simulink model "transientStability_R14SP1"  (Simulink 6.1)
settings: Solver=ode4  SolverMode=SingleTasking  StartTime=0.0  StopTime=10  FixedStep=0.01  MaxStep=0.01  RelTol=1e-3  AbsTol=1e-2
undefined symbols (not defined in the file): j, mpc
(part 2 of 3)

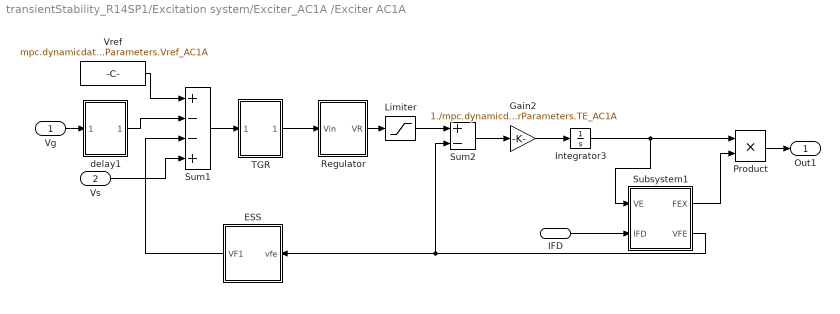
== system transientStability_R14SP1/Excitation system/Exciter_AC1A /Exciter AC1A ==
  Vg : Inport
  Vs : Inport  Port=2
  IFD : Inport  Port=3
  ESS : Subsystem  Orientation=left
  Gain2 : Gain  Gain=1./mpc.dynamicdata.gen_exciterParameters.AC1A_exciterParameters.TE_AC1A  SaturateOnIntegerOverflow=on
  Integrator3 : Integrator  InitialCondition=mpc.dynamicdata.gen_exciterParameters.AC1A_exciterParameters.Ve_AC1A  LimitOutput=on  LowerSaturationLimit=0.01
  Limiter : Saturate  UpperLimit=mpc.dynamicdata.gen_exciterParameters.AC1A_exciterParameters.VRmax_AC1A  LowerLimit=mpc.dynamicdata.gen_exciterParameters.AC1A_exciterParameters.VRmin_AC1A
  Product : Product  SaturateOnIntegerOverflow=on  RndMeth=Zero  InputSameDT=on
  Regulator : Subsystem
  Subsystem1 : Subsystem
  Sum1 : Sum  Inputs=+--+  SaturateOnIntegerOverflow=on  InputSameDT=on
  Sum2 : Sum  Inputs=+-  SaturateOnIntegerOverflow=on  InputSameDT=on
  TGR : Subsystem
  Vref : Constant  Value=mpc.dynamicdata.gen_exciterParameters.AC1A_exciterParameters.Vref_AC1A
  delay1 : Subsystem
  Out1 : Outport
  wires:
  Regulator/1(VR) -> Limiter/1
  Sum1/1 -> TGR/1(Ver)
  TGR/1(Vtgr) -> Regulator/1(Vin)
  Vref/1 -> Sum1/1
  Vs/1 -> Sum1/4
  Product/1 -> Out1/1
  IFD/1 -> Subsystem1/2(IFD)
  Sum2/1 -> Gain2/1
  Limiter/1 -> Sum2/1
  ESS/1(VF1) -> Sum1/3
  Gain2/1 -> Integrator3/1
  Subsystem1/1(FEX) -> Product/2
  Subsystem1/2(VFE) -> ESS/1(vfe), Sum2/2
  Integrator3/1 -> Subsystem1/1(VE), Product/1
  delay1/1(Out1) -> Sum1/2
  Vg/1 -> delay1/1(Vin)

== system transientStability_R14SP1/Excitation system/Exciter_AC1A /Select-AVR ==
  in_1 : Inport
  in_2 : Inport  Port=2
  Switch : Switch  Threshold=1  SaturateOnIntegerOverflow=on  InputSameDT=on
  zeros : Constant  Value=zeros(1,mpc.dynamicdata.extraVariables.nb)
  out_1 : Outport  InitialOutput=0
  wires:
  in_2/1 -> Switch/3
  in_1/1 -> Switch/2
  Switch/1 -> out_1/1
  zeros/1 -> Switch/1

== system transientStability_R14SP1/Excitation system/Exciter_AC4A/DEMUXg2 ==
  In1 : Inport
  Dummy Zeros : Constant  Value=zeros(1,mpc.dynamicdata.extraVariables.nb-size(mpc.dynamicdata.exc_AC4A,1))
  Mux1 : Mux  Inputs="[mpc.dynamicdata.extraVariables.nb-size(mpc.dynamicdata.exc_AC4A,1)  size(mpc.dynamicdata.exc_AC4A,1)]"
  Selector4 : Selector  InputPortWidth=mpc.dynamicdata.extraVariables.nb
  Out1 : Outport
  wires:
  In1/1 -> Mux1/2
  Selector4/1 -> Out1/1
  Dummy Zeros/1 -> Mux1/1
  Mux1/1 -> Selector4/1

== system transientStability_R14SP1/Excitation system/Exciter_AC4A/Exciter_AC4A ==
  Vg : Inport
  Vs : Inport  Port=2
  IFD : Inport  Port=3
  REG : Subsystem
  Saturation : Saturate  UpperLimit=mpc.dynamicdata.gen_exciterParameters.AC4A_exciterParameters.VImax_AC4A  LowerLimit=mpc.dynamicdata.gen_exciterParameters.AC4A_exciterParameters.VImin_AC4A
  Sum1 : Sum  Inputs=+-+  SaturateOnIntegerOverflow=on  InputSameDT=on
  TGR : Subsystem
  Vref1 : Constant  Value=mpc.dynamicdata.gen_exciterParameters.AC4A_exciterParameters.Vref_AC4A
  delay1 : Subsystem
  Out1 : Outport
  wires:
  TGR/1(V3) -> REG/1(In1)
  Vref1/1 -> Sum1/1
  Vs/1 -> Sum1/3
  IFD/1 -> REG/2(IFD)
  REG/1(Out1) -> Out1/1
  Sum1/1 -> Saturation/1
  Saturation/1 -> TGR/1(Ver)
  Vg/1 -> delay1/1(Vin)
  delay1/1(Out1) -> Sum1/2

== system transientStability_R14SP1/Excitation system/Exciter_AC4A/Select-AVR ==
  in_1 : Inport
  in_2 : Inport  Port=2
  Switch : Switch  Threshold=1  SaturateOnIntegerOverflow=on  InputSameDT=on
  zeros : Constant  Value=zeros(1,mpc.dynamicdata.extraVariables.nb)
  out_1 : Outport  InitialOutput=0
  wires:
  in_2/1 -> Switch/3
  in_1/1 -> Switch/2
  Switch/1 -> out_1/1
  zeros/1 -> Switch/1

== system transientStability_R14SP1/Excitation system/Exciter_DC1A/DEMUXg2 ==
  In1 : Inport
  Dummy Zeros : Constant  Value=zeros(1,mpc.dynamicdata.extraVariables.nb-size(mpc.dynamicdata.exc_DC1A,1))
  Mux1 : Mux  Inputs="[mpc.dynamicdata.extraVariables.nb-size(mpc.dynamicdata.exc_DC1A,1)  size(mpc.dynamicdata.exc_DC1A,1)]"
  Selector4 : Selector  InputPortWidth=mpc.dynamicdata.extraVariables.nb
  Out1 : Outport
  wires:
  In1/1 -> Mux1/2
  Selector4/1 -> Out1/1
  Dummy Zeros/1 -> Mux1/1
  Mux1/1 -> Selector4/1

== system transientStability_R14SP1/Excitation system/Exciter_DC1A/Select-AVR ==
  in_1 : Inport
  in_2 : Inport  Port=2
  Switch : Switch  Threshold=1  SaturateOnIntegerOverflow=on  InputSameDT=on
  zeros : Constant  Value=zeros(1,mpc.dynamicdata.extraVariables.nb)
  out_1 : Outport  InitialOutput=0
  wires:
  in_2/1 -> Switch/3
  in_1/1 -> Switch/2
  Switch/1 -> out_1/1
  zeros/1 -> Switch/1

== system transientStability_R14SP1/Excitation system/Exciter_DC1A/Subsystem ==
  Vg : Inport
  Vs : Inport  Port=2
  ESS : Subsystem  Orientation=left
  Gain2 : Gain  Gain=1./mpc.dynamicdata.gen_exciterParameters.DC1A_exciterParameters.TE_DC1A  SaturateOnIntegerOverflow=on
  Integrator3 : Integrator  InitialCondition=mpc.dynamicdata.gen_exciterParameters.DC1A_exciterParameters.Efd0_DC1A
  Regulator : Subsystem
  Saturation : Subsystem  Orientation=left
  Sum1 : Sum  Inputs=+--+  SaturateOnIntegerOverflow=on  InputSameDT=on
  Sum2 : Sum  Inputs=+-  SaturateOnIntegerOverflow=on  InputSameDT=on
  TGR : Subsystem
  Vref : Constant  Value=mpc.dynamicdata.gen_exciterParameters.DC1A_exciterParameters.Vref_DC1A
  delay1 : Subsystem
  Efd : Outport
  wires:
  ESS/1(VF) -> Sum1/3
  Sum1/1 -> TGR/1(Ver)
  TGR/1(V3) -> Regulator/1(Vin)
  Sum2/1 -> Gain2/1
  Gain2/1 -> Integrator3/1
  Saturation/1(VRb) -> Sum2/2
  Integrator3/1 -> Saturation/1(Efd), ESS/1(Efd), Efd/1
  Vs/1 -> Sum1/4
  Vref/1 -> Sum1/1
  delay1/1(Out1) -> Sum1/2
  Vg/1 -> delay1/1(Vin)
  Regulator/1(Out1) -> Sum2/1

== system transientStability_R14SP1/Excitation system/Exciter_ST1A/DEMUXg2 ==
  In1 : Inport
  Dummy Zeros : Constant  Value=zeros(1,mpc.dynamicdata.extraVariables.nb-size(mpc.dynamicdata.exc_ST1A,1))
  Mux1 : Mux  Inputs="[mpc.dynamicdata.extraVariables.nb-size(mpc.dynamicdata.exc_ST1A,1)  size(mpc.dynamicdata.exc_ST1A,1)]"
  Selector4 : Selector  InputPortWidth=mpc.dynamicdata.extraVariables.nb
  Out1 : Outport
  wires:
  In1/1 -> Mux1/2
  Selector4/1 -> Out1/1
  Dummy Zeros/1 -> Mux1/1
  Mux1/1 -> Selector4/1

== system transientStability_R14SP1/Excitation system/Exciter_ST1A/Select-AVR ==
  in_1 : Inport
  in_2 : Inport  Port=2
  Switch : Switch  Threshold=1  SaturateOnIntegerOverflow=on  InputSameDT=on
  zeros : Constant  Value=zeros(1,mpc.dynamicdata.extraVariables.nb)
  out_1 : Outport  InitialOutput=0
  wires:
  in_2/1 -> Switch/3
  in_1/1 -> Switch/2
  Switch/1 -> out_1/1
  zeros/1 -> Switch/1

== system transientStability_R14SP1/Excitation system/Exciter_ST1A/delay1 ==
  Vin : Inport
  Gain : Gain  Gain=1./mpc.dynamicdata.gen_exciterParameters.ST1A_exciterParameters.Tr_ST1A  SaturateOnIntegerOverflow=on
  Integrator2 : Integrator  InitialCondition=mpc.dynamicdata.extraVariables.lfl(mpc.dynamicdata.exc_ST1A(:,1),2)
  Sum : Sum  Inputs=+-  SaturateOnIntegerOverflow=on  InputSameDT=on
  Out1 : Outport
  wires:
  Vin/1 -> Sum/1
  Integrator2/1 -> Sum/2, Out1/1
  Sum/1 -> Gain/1
  Gain/1 -> Integrator2/1

== system transientStability_R14SP1/Excitation system/Exciter_ST1A/exc_ST1A ==
  Vg : Inport
  Vs : Inport  Port=2
  IFD : Inport  Port=3
  ESS : Subsystem  Orientation=left
  Gain2 : Gain  Gain=mpc.dynamicdata.gen_exciterParameters.ST1A_exciterParameters.KLR_ST1A  SaturateOnIntegerOverflow=on
  ILR : Constant  Value=mpc.dynamicdata.gen_exciterParameters.ST1A_exciterParameters.ILR_ST1A
  Limiter : Subsystem
  Rergulator : Subsystem
  Saturation1 : Saturate  UpperLimit=inf  LowerLimit=0
  Sum1 : Sum  Inputs=+-+-  SaturateOnIntegerOverflow=on  InputSameDT=on
  Sum2 : Sum  Inputs=+-  SaturateOnIntegerOverflow=on  InputSameDT=on
  Sum3 : Sum  Inputs=+-  SaturateOnIntegerOverflow=on  InputSameDT=on
  TGR : Subsystem
  Vref1 : Constant  Value=mpc.dynamicdata.gen_exciterParameters.ST1A_exciterParameters.Vref_ST1A
  out_1 : Outport  InitialOutput=0
  wires:
  Vref1/1 -> Sum1/1
  Vs/1 -> Sum1/3
  Rergulator/1(Out1) -> Sum3/1
  Vg/1 -> Sum1/2, Limiter/3(Vt)
  Limiter/1(Out1) -> out_1/1
  ILR/1 -> Sum2/2
  Sum2/1 -> Gain2/1
  Gain2/1 -> Saturation1/1
  Saturation1/1 -> Sum3/2
  IFD/1 -> Sum2/1, Limiter/2(IFD)
  Sum1/1 -> TGR/1(Ver)
  TGR/1(V3) -> Rergulator/1(In1)
  Sum3/1 -> Limiter/1(In1), ESS/1(Efd)
  ESS/1(VF) -> Sum1/4

== system transientStability_R14SP1/Excitation system/Exciter_ST2A/DEMUXg2 ==
  In1 : Inport
  Dummy Zeros : Constant  Value=zeros(1,mpc.dynamicdata.extraVariables.nb-size(mpc.dynamicdata.exc_ST2A,1))
  Mux1 : Mux  Inputs="[mpc.dynamicdata.extraVariables.nb-size(mpc.dynamicdata.exc_ST2A,1)  size(mpc.dynamicdata.exc_ST2A,1)]"
  Selector4 : Selector  InputPortWidth=mpc.dynamicdata.extraVariables.nb
  Out1 : Outport
  wires:
  Mux1/1 -> Selector4/1
  Dummy Zeros/1 -> Mux1/1
  Selector4/1 -> Out1/1
  In1/1 -> Mux1/2

== system transientStability_R14SP1/Excitation system/Exciter_ST2A/ST2A_Exciter ==
  IFD : Inport
  Ia : Inport  Port=2
  Vg : Inport  Port=3
  Vs : Inport  Port=4
  Comp to Mag : ComplexToMagnitudeAngle
  ESS : Subsystem  Orientation=left
  Product4 : Product  SaturateOnIntegerOverflow=on  RndMeth=Zero  InputSameDT=on
  Regulator : Subsystem
  Subsystem : Subsystem
  Sum2 : Sum  Inputs=+--+  SaturateOnIntegerOverflow=on  InputSameDT=on
  Term : Terminator
      settings: Orientation=down
  Vref : Constant  Value=mpc.dynamicdata.gen_exciterParameters.ST2A_exciterParameters.Vref_ST2A
  exciter : Subsystem
  Efd : Outport
  wires:
  Sum2/1 -> Regulator/1(Vin)
  ESS/1(VF) -> Sum2/3
  Vs/1 -> Sum2/4
  Vref/1 -> Sum2/1
  exciter/1(Out1) -> ESS/1(EFD), Efd/1
  IFD/1 -> Subsystem/2("IFD ")
  Ia/1 -> Subsystem/3(Ia)
  Subsystem/1(VB) -> Product4/2
  Product4/1 -> exciter/1(In1)
  Vg/1 -> Subsystem/1(VT), Comp to Mag/1
  Comp to Mag/2 -> Term/1
  Comp to Mag/1 -> Sum2/2
  Regulator/1(Out1) -> Product4/1

== system transientStability_R14SP1/Excitation system/Exciter_ST2A/Select-AVR ==
  in_1 : Inport
  in_2 : Inport  Port=2
  Switch : Switch  Threshold=1  SaturateOnIntegerOverflow=on  InputSameDT=on
  zeros : Constant  Value=zeros(1,mpc.dynamicdata.extraVariables.nb)
  out_1 : Outport  InitialOutput=0
  wires:
  in_2/1 -> Switch/3
  in_1/1 -> Switch/2
  Switch/1 -> out_1/1
  zeros/1 -> Switch/1

== system transientStability_R14SP1/Excitation system/Exciter_static/DEMUXg2 ==
  In1 : Inport
  Dummy Zeros : Constant  Value=zeros(1,mpc.dynamicdata.extraVariables.nb-size(mpc.dynamicdata.exc_static,1))
  Mux1 : Mux  Inputs="[mpc.dynamicdata.extraVariables.nb-size(mpc.dynamicdata.exc_static,1)  size(mpc.dynamicdata.exc_static,1)]"
  Selector4 : Selector  InputPortWidth=mpc.dynamicdata.extraVariables.nb
  Out1 : Outport
  wires:
  In1/1 -> Mux1/2
  Selector4/1 -> Out1/1
  Dummy Zeros/1 -> Mux1/1
  Mux1/1 -> Selector4/1

== system transientStability_R14SP1/Excitation system/Exciter_static/Select-AVR ==
  in_1 : Inport
  in_2 : Inport  Port=2
  Switch : Switch  Threshold=1  SaturateOnIntegerOverflow=on  InputSameDT=on
  zeros : Constant  Value=zeros(1,mpc.dynamicdata.extraVariables.nb)
  out_1 : Outport  InitialOutput=0
  wires:
  in_2/1 -> Switch/3
  in_1/1 -> Switch/2
  Switch/1 -> out_1/1
  zeros/1 -> Switch/1

== system transientStability_R14SP1/Excitation system/Exciter_static/exc_static ==
  Vg : Inport
  Vs : Inport  Port=2
  Gain : Gain  Gain=1./mpc.dynamicdata.gen_exciterParameters.static_exciterParameters.TA_static  SaturateOnIntegerOverflow=on
  Gain1 : Gain  Gain=mpc.dynamicdata.gen_exciterParameters.static_exciterParameters.kA_static  SaturateOnIntegerOverflow=on
  Integrator2 : Integrator  InitialCondition=mpc.dynamicdata.gen_exciterParameters.static_exciterParameters.Efd0_static
  Saturation : Saturate  UpperLimit=mpc.dynamicdata.gen_exciterParameters.static_exciterParameters.Efd_max_static  LowerLimit=mpc.dynamicdata.gen_exciterParameters.static_exciterParameters.Efd_min_static
  Sum : Sum  Inputs=+-  SaturateOnIntegerOverflow=on  InputSameDT=on
  Sum1 : Sum  Inputs=+-+  SaturateOnIntegerOverflow=on  InputSameDT=on
  Vref1 : Constant  Value=mpc.dynamicdata.gen_exciterParameters.static_exciterParameters.Vref_static
  out_1 : Outport  InitialOutput=0
  wires:
  Gain/1 -> Integrator2/1
  Integrator2/1 -> Saturation/1, Sum/2
  Saturation/1 -> out_1/1
  Vg/1 -> Sum1/2
  Sum1/1 -> Gain1/1
  Sum/1 -> Gain/1
  Gain1/1 -> Sum/1
  Vref1/1 -> Sum1/1
  Vs/1 -> Sum1/3

== system transientStability_R14SP1/PSS/PSS_slip_signal/Compensator ==
  in : Inport
  Gain3 : Gain  Gain=1./mpc.dynamicdata.gen_pssParameters.pss_slip_signalParameters.T2_slip  SaturateOnIntegerOverflow=on
  Gain4 : Gain  Gain=mpc.dynamicdata.gen_pssParameters.pss_slip_signalParameters.T1_slip./mpc.dynamicdata.gen_pssParameters.pss_slip_signalParameters.T2_slip  SaturateOnIntegerOverflow=on
  Gain5 : Gain  Gain=1-mpc.dynamicdata.gen_pssParameters.pss_slip_signalParameters.T1_slip./mpc.dynamicdata.gen_pssParameters.pss_slip_signalParameters.T2_slip  SaturateOnIntegerOverflow=on
  Integrator4 : Integrator
  Sum3 : Sum  SaturateOnIntegerOverflow=on  InputSameDT=on
  Sum4 : Sum  Inputs=+-  SaturateOnIntegerOverflow=on  InputSameDT=on
  Vs : Outport
  wires:
  Gain5/1 -> Sum4/1
  Sum4/1 -> Gain3/1
  Gain3/1 -> Integrator4/1
  Integrator4/1 -> Sum4/2, Sum3/1
  Gain4/1 -> Sum3/2
  in/1 -> Gain5/1, Gain4/1
  Sum3/1 -> Vs/1

== system transientStability_R14SP1/PSS/PSS_slip_signal/DEMUXg2 ==
  In1 : Inport
  Dummy Zeros : Constant  Value=zeros(1,mpc.dynamicdata.extraVariables.nb-size(mpc.dynamicdata.slip_pss,1))
  Mux1 : Mux  Inputs="[mpc.dynamicdata.extraVariables.nb-size(mpc.dynamicdata.slip_pss,1)  size(mpc.dynamicdata.slip_pss,1)]"
  Selector4 : Selector  InputPortWidth=mpc.dynamicdata.extraVariables.nb
  Out1 : Outport
  wires:
  In1/1 -> Mux1/2
  Selector4/1 -> Out1/1
  Dummy Zeros/1 -> Mux1/1
  Mux1/1 -> Selector4/1

== system transientStability_R14SP1/PSS/PSS_slip_signal/FILT(s) ==
  In1 : Inport
  Gain : Gain  Gain=570  SaturateOnIntegerOverflow=on
  Gain1 : Gain  Orientation=left  Gain=35  SaturateOnIntegerOverflow=on
  Gain2 : Gain  Orientation=left  Gain=570  SaturateOnIntegerOverflow=on
  Integrator : Integrator
  Integrator1 : Integrator
  Sum : Sum  Inputs=|+--  SaturateOnIntegerOverflow=on  InputSameDT=on
  Vs : Outport
  wires:
  Gain/1 -> Sum/1
  Sum/1 -> Integrator/1
  Integrator/1 -> Integrator1/1, Gain1/1
  Gain1/1 -> Sum/3
  Gain2/1 -> Sum/2
  Integrator1/1 -> Gain2/1, Vs/1
  In1/1 -> Gain/1

== system transientStability_R14SP1/PSS/PSS_slip_signal/Select-PSS ==
  in_1 : Inport
  in_2 : Inport  Port=2
  Switch : Switch  Threshold=1  SaturateOnIntegerOverflow=on  InputSameDT=on
  Vs=0 : Constant  Value=zeros(1,mpc.dynamicdata.extraVariables.nb)
  out_1 : Outport  InitialOutput=0
  wires:
  in_2/1 -> Switch/3
  in_1/1 -> Switch/2
  Switch/1 -> out_1/1
  Vs=0/1 -> Switch/1

== system transientStability_R14SP1/PSS/PSS_slip_signal/Wash_out ==
  in : Inport
  Gain3 : Gain  Gain=1./mpc.dynamicdata.gen_pssParameters.pss_slip_signalParameters.Tw_slip  SaturateOnIntegerOverflow=on
  Gain4 : Gain  Gain=mpc.dynamicdata.gen_pssParameters.pss_slip_signalParameters.Tw_slip  SaturateOnIntegerOverflow=on
  Integrator4 : Integrator
  Sum3 : Sum  Inputs=+-  SaturateOnIntegerOverflow=on  InputSameDT=on
  out : Outport  Orientation=up
  wires:
  Gain4/1 -> Sum3/1
  Sum3/1 -> Gain3/1
  Integrator4/1 -> Sum3/2
  Gain3/1 -> Integrator4/1, out/1
  in/1 -> Gain4/1

== system transientStability_R14SP1/PSS/PSS_slip_signal/delay ==
  Vin : Inport
  Gain : Gain  Gain=1./mpc.dynamicdata.gen_pssParameters.pss_slip_signalParameters.Td1_slip  SaturateOnIntegerOverflow=on
  Integrator2 : Integrator
  Sum : Sum  Inputs=+-  SaturateOnIntegerOverflow=on  InputSameDT=on
  Out1 : Outport
  wires:
  Gain/1 -> Integrator2/1
  Sum/1 -> Gain/1
  Integrator2/1 -> Out1/1, Sum/2
  Vin/1 -> Sum/1

== system transientStability_R14SP1/PSS/Power_input_PSS/DEMUXg2 ==
  In1 : Inport
  Dummy Zeros : Constant  Value=zeros(1,mpc.dynamicdata.extraVariables.nb-size(mpc.dynamicdata.power_pss,1))
  Mux1 : Mux  Inputs="[mpc.dynamicdata.extraVariables.nb-size(mpc.dynamicdata.power_pss,1)  size(mpc.dynamicdata.power_pss,1)]"
  Selector4 : Selector  InputPortWidth=mpc.dynamicdata.extraVariables.nb
  Out1 : Outport
  wires:
  Mux1/1 -> Selector4/1
  Dummy Zeros/1 -> Mux1/1
  Selector4/1 -> Out1/1
  In1/1 -> Mux1/2

== system transientStability_R14SP1/PSS/Power_input_PSS/Select-PSS ==
  in_1 : Inport
  in_2 : Inport  Port=2
  Switch : Switch  Threshold=1  SaturateOnIntegerOverflow=on  InputSameDT=on
  Vs=0 : Constant  Value=zeros(1,mpc.dynamicdata.extraVariables.nb)
  out_1 : Outport  InitialOutput=0
  wires:
  in_2/1 -> Switch/3
  in_1/1 -> Switch/2
  Switch/1 -> out_1/1
  Vs=0/1 -> Switch/1

== system transientStability_R14SP1/PSS/Power_input_PSS/Wash_out ==
  in : Inport
  Gain3 : Gain  Gain=1./mpc.dynamicdata.gen_pssParameters.pss_power_signalParameters.Tw_power  SaturateOnIntegerOverflow=on
  Gain4 : Gain  Gain=mpc.dynamicdata.gen_pssParameters.pss_power_signalParameters.Tw_power  SaturateOnIntegerOverflow=on
  Integrator4 : Integrator  InitialCondition=mpc.dynamicdata.gen_pssParameters.pss_power_signalParameters.Tm0_power.*mpc.dynamicdata.gen_pssParameters.pss_power_signalParameters.Tw_power
  Sum3 : Sum  Inputs=+-  SaturateOnIntegerOverflow=on  InputSameDT=on
  out : Outport  Orientation=up
  wires:
  in/1 -> Gain4/1
  Gain3/1 -> out/1, Integrator4/1
  Integrator4/1 -> Sum3/2
  Sum3/1 -> Gain3/1
  Gain4/1 -> Sum3/1

== system transientStability_R14SP1/PSS/Power_input_PSS/delay1 ==
  Vin : Inport
  Gain : Gain  Gain=1./mpc.dynamicdata.gen_pssParameters.pss_power_signalParameters.Td1_power  SaturateOnIntegerOverflow=on
  Integrator2 : Integrator
  Sum : Sum  Inputs=+-  SaturateOnIntegerOverflow=on  InputSameDT=on
  Out1 : Outport
  wires:
  Vin/1 -> Sum/1
  Integrator2/1 -> Sum/2, Out1/1
  Sum/1 -> Gain/1
  Gain/1 -> Integrator2/1

== system transientStability_R14SP1/PSS/delP_Omega_PSS/Compensator ==
  in : Inport
  Gain3 : Gain  Gain=1./mpc.dynamicdata.gen_pssParameters.pss_delPw_signalParameters.T2_delPw  SaturateOnIntegerOverflow=on
  Gain4 : Gain  Gain=mpc.dynamicdata.gen_pssParameters.pss_delPw_signalParameters.T1_delPw./mpc.dynamicdata.gen_pssParameters.pss_delPw_signalParameters.T2_delPw  SaturateOnIntegerOverflow=on
  Gain5 : Gain  Gain=1-mpc.dynamicdata.gen_pssParameters.pss_delPw_signalParameters.T1_delPw./mpc.dynamicdata.gen_pssParameters.pss_delPw_signalParameters.T2_delPw  SaturateOnIntegerOverflow=on
  Integrator4 : Integrator
  Sum3 : Sum  SaturateOnIntegerOverflow=on  InputSameDT=on
  Sum4 : Sum  Inputs=+-  SaturateOnIntegerOverflow=on  InputSameDT=on
  Vs : Outport
  wires:
  Gain5/1 -> Sum4/1
  Sum4/1 -> Gain3/1
  Gain3/1 -> Integrator4/1
  Integrator4/1 -> Sum4/2, Sum3/1
  Gain4/1 -> Sum3/2
  in/1 -> Gain5/1, Gain4/1
  Sum3/1 -> Vs/1

== system transientStability_R14SP1/PSS/delP_Omega_PSS/DEMUXg2 ==
  In1 : Inport
  Dummy Zeros : Constant  Value=zeros(1,mpc.dynamicdata.extraVariables.nb-size(mpc.dynamicdata.delPw_pss,1))
  Mux1 : Mux  Inputs="[mpc.dynamicdata.extraVariables.nb-size(mpc.dynamicdata.delPw_pss,1)  size(mpc.dynamicdata.delPw_pss,1)]"
  Selector4 : Selector  InputPortWidth=mpc.dynamicdata.extraVariables.nb
  Out1 : Outport
  wires:
  Mux1/1 -> Selector4/1
  Dummy Zeros/1 -> Mux1/1
  Selector4/1 -> Out1/1
  In1/1 -> Mux1/2

== system transientStability_R14SP1/PSS/delP_Omega_PSS/Filtering M=2 and N=4 ==
  note: M=2 and N=4
  In1 : Inport
  Subsystem : Subsystem
  Subsystem1 : Subsystem
  Subsystem2 : Subsystem
  Subsystem3 : Subsystem
  Out1 : Outport
  wires:
  Subsystem2/1(Out2) -> Subsystem3/1(In1)
  Subsystem1/1(Out2) -> Subsystem2/1(In1)
  Subsystem/1(Out2) -> Subsystem1/1(In1)
  Subsystem3/1(Out2) -> Out1/1
  In1/1 -> Subsystem/1(In1)

== system transientStability_R14SP1/PSS/delP_Omega_PSS/Integrator ==
  Vin : Inport
  Gain : Gain  Gain=1./mpc.dynamicdata.gen_pssParameters.pss_delPw_signalParameters.T7_delPw  SaturateOnIntegerOverflow=on
  Gain1 : Gain  Gain=mpc.dynamicdata.gen_pssParameters.pss_delPw_signalParameters.T7_delPw./(2*mpc.dynamicdata.gen_pssParameters.pss_delPw_signalParameters.H_delPw)  SaturateOnIntegerOverflow=on
  Integrator2 : Integrator
  Sum : Sum  Inputs=+-  SaturateOnIntegerOverflow=on  InputSameDT=on
  Out1 : Outport
  wires:
  Gain1/1 -> Sum/1
  Integrator2/1 -> Sum/2, Out1/1
  Sum/1 -> Gain/1
  Gain/1 -> Integrator2/1
  Vin/1 -> Gain1/1

== system transientStability_R14SP1/PSS/delP_Omega_PSS/Select-PSS ==
  in_1 : Inport
  in_2 : Inport  Port=2
  Switch : Switch  Threshold=1  SaturateOnIntegerOverflow=on  InputSameDT=on
  Vs=0 : Constant  Value=zeros(1,mpc.dynamicdata.extraVariables.nb)
  out_1 : Outport  InitialOutput=0
  wires:
  in_2/1 -> Switch/3
  in_1/1 -> Switch/2
  Switch/1 -> out_1/1
  Vs=0/1 -> Switch/1

== system transientStability_R14SP1/PSS/delP_Omega_PSS/Wash_out_1 ==
  in : Inport
  Gain3 : Gain  Gain=1./mpc.dynamicdata.gen_pssParameters.pss_delPw_signalParameters.Tw1_delPw  SaturateOnIntegerOverflow=on
  Gain4 : Gain  Gain=mpc.dynamicdata.gen_pssParameters.pss_delPw_signalParameters.Tw1_delPw  SaturateOnIntegerOverflow=on
  Integrator4 : Integrator
  Sum3 : Sum  Inputs=+-  SaturateOnIntegerOverflow=on  InputSameDT=on
  out : Outport  Orientation=up
  wires:
  Gain4/1 -> Sum3/1
  Sum3/1 -> Gain3/1
  Integrator4/1 -> Sum3/2
  Gain3/1 -> Integrator4/1, out/1
  in/1 -> Gain4/1

== system transientStability_R14SP1/PSS/delP_Omega_PSS/Wash_out_2 ==
  in : Inport
  Gain3 : Gain  Gain=1./mpc.dynamicdata.gen_pssParameters.pss_delPw_signalParameters.Tw2_delPw  SaturateOnIntegerOverflow=on
  Gain4 : Gain  Gain=mpc.dynamicdata.gen_pssParameters.pss_delPw_signalParameters.Tw2_delPw  SaturateOnIntegerOverflow=on
  Integrator4 : Integrator
  Sum3 : Sum  Inputs=+-  SaturateOnIntegerOverflow=on  InputSameDT=on
  out : Outport  Orientation=up
  wires:
  in/1 -> Gain4/1
  Gain3/1 -> out/1, Integrator4/1
  Integrator4/1 -> Sum3/2
  Sum3/1 -> Gain3/1
  Gain4/1 -> Sum3/1

== system transientStability_R14SP1/PSS/delP_Omega_PSS/Wash_out_3 ==
  in : Inport
  Gain3 : Gain  Gain=1./mpc.dynamicdata.gen_pssParameters.pss_delPw_signalParameters.Tw3_delPw  SaturateOnIntegerOverflow=on
  Gain4 : Gain  Gain=mpc.dynamicdata.gen_pssParameters.pss_delPw_signalParameters.Tw3_delPw  SaturateOnIntegerOverflow=on
  Integrator4 : Integrator  InitialCondition=mpc.dynamicdata.gen_pssParameters.pss_delPw_signalParameters.Tm0_delPw.*mpc.dynamicdata.gen_pssParameters.pss_delPw_signalParameters.Tw3_delPw
  Sum3 : Sum  Inputs=+-  SaturateOnIntegerOverflow=on  InputSameDT=on
  out : Outport  Orientation=up
  wires:
  in/1 -> Gain4/1
  Gain3/1 -> out/1, Integrator4/1
  Integrator4/1 -> Sum3/2
  Sum3/1 -> Gain3/1
  Gain4/1 -> Sum3/1

== system transientStability_R14SP1/PSS/delP_Omega_PSS/Wash_out_4 ==
  in : Inport
  Gain3 : Gain  Gain=1./mpc.dynamicdata.gen_pssParameters.pss_delPw_signalParameters.Tw4_delPw  SaturateOnIntegerOverflow=on
  Gain4 : Gain  Gain=mpc.dynamicdata.gen_pssParameters.pss_delPw_signalParameters.Tw4_delPw  SaturateOnIntegerOverflow=on
  Integrator4 : Integrator
  Sum3 : Sum  Inputs=+-  SaturateOnIntegerOverflow=on  InputSameDT=on
  out : Outport  Orientation=up
  wires:
  Gain4/1 -> Sum3/1
  Sum3/1 -> Gain3/1
  Integrator4/1 -> Sum3/2
  Gain3/1 -> Integrator4/1, out/1
  in/1 -> Gain4/1

== system transientStability_R14SP1/PSS/delP_Omega_PSS/delay ==
  Vin : Inport
  Gain : Gain  Gain=1./mpc.dynamicdata.gen_pssParameters.pss_delPw_signalParameters.T6_delPw  SaturateOnIntegerOverflow=on
  Integrator2 : Integrator
  Sum : Sum  Inputs=+-  SaturateOnIntegerOverflow=on  InputSameDT=on
  Out1 : Outport
  wires:
  Gain/1 -> Integrator2/1
  Sum/1 -> Gain/1
  Integrator2/1 -> Out1/1, Sum/2
  Vin/1 -> Sum/1

== system transientStability_R14SP1/PSS/frequency_input_PSS /Compensator ==
  in : Inport
  Gain3 : Gain  Gain=1./mpc.dynamicdata.gen_pssParameters.pss_freq_signalParameters.T2_freq  SaturateOnIntegerOverflow=on
  Gain4 : Gain  Gain=mpc.dynamicdata.gen_pssParameters.pss_freq_signalParameters.T1_freq./mpc.dynamicdata.gen_pssParameters.pss_freq_signalParameters.T2_freq  SaturateOnIntegerOverflow=on
  Gain5 : Gain  Gain=1-mpc.dynamicdata.gen_pssParameters.pss_freq_signalParameters.T1_freq./mpc.dynamicdata.gen_pssParameters.pss_freq_signalParameters.T2_freq  SaturateOnIntegerOverflow=on
  Integrator4 : Integrator
  Sum3 : Sum  SaturateOnIntegerOverflow=on  InputSameDT=on
  Sum4 : Sum  Inputs=+-  SaturateOnIntegerOverflow=on  InputSameDT=on
  Vs : Outport
  wires:
  Gain5/1 -> Sum4/1
  Sum4/1 -> Gain3/1
  Gain3/1 -> Integrator4/1
  Integrator4/1 -> Sum4/2, Sum3/1
  Gain4/1 -> Sum3/2
  in/1 -> Gain5/1, Gain4/1
  Sum3/1 -> Vs/1

== system transientStability_R14SP1/PSS/frequency_input_PSS /DEMUXg2 ==
  In1 : Inport
  Dummy Zeros : Constant  Value=zeros(1,mpc.dynamicdata.extraVariables.nb-size(mpc.dynamicdata.freq_pss,1))
  Mux1 : Mux  Inputs="[mpc.dynamicdata.extraVariables.nb-size(mpc.dynamicdata.freq_pss,1)  size(mpc.dynamicdata.freq_pss,1)]"
  Selector4 : Selector  InputPortWidth=mpc.dynamicdata.extraVariables.nb
  Out1 : Outport
  wires:
  Mux1/1 -> Selector4/1
  Dummy Zeros/1 -> Mux1/1
  Selector4/1 -> Out1/1
  In1/1 -> Mux1/2

== system transientStability_R14SP1/PSS/frequency_input_PSS /FILT(s) ==
  In1 : Inport
  Gain : Gain  Gain=570  SaturateOnIntegerOverflow=on
  Gain1 : Gain  Orientation=left  Gain=35  SaturateOnIntegerOverflow=on
  Gain2 : Gain  Orientation=left  Gain=570  SaturateOnIntegerOverflow=on
  Integrator : Integrator
  Integrator1 : Integrator
  Sum : Sum  Inputs=|+--  SaturateOnIntegerOverflow=on  InputSameDT=on
  Vs : Outport
  wires:
  Gain/1 -> Sum/1
  Sum/1 -> Integrator/1
  Integrator/1 -> Integrator1/1, Gain1/1
  Gain1/1 -> Sum/3
  Gain2/1 -> Sum/2
  Integrator1/1 -> Gain2/1, Vs/1
  In1/1 -> Gain/1

== system transientStability_R14SP1/PSS/frequency_input_PSS /Select-PSS ==
  in_1 : Inport
  in_2 : Inport  Port=2
  Switch : Switch  Threshold=1  SaturateOnIntegerOverflow=on  InputSameDT=on
  Vs=0 : Constant  Value=zeros(1,mpc.dynamicdata.extraVariables.nb)
  out_1 : Outport  InitialOutput=0
  wires:
  in_2/1 -> Switch/3
  in_1/1 -> Switch/2
  Switch/1 -> out_1/1
  Vs=0/1 -> Switch/1

== system transientStability_R14SP1/PSS/frequency_input_PSS /Wash_out ==
  in : Inport
  Gain3 : Gain  Gain=1./mpc.dynamicdata.gen_pssParameters.pss_freq_signalParameters.Tw_freq  SaturateOnIntegerOverflow=on
  Gain4 : Gain  Gain=mpc.dynamicdata.gen_pssParameters.pss_freq_signalParameters.Tw_freq  SaturateOnIntegerOverflow=on
  Integrator4 : Integrator
  Sum3 : Sum  Inputs=+-  SaturateOnIntegerOverflow=on  InputSameDT=on
  out : Outport  Orientation=up
  wires:
  in/1 -> Gain4/1
  Gain3/1 -> out/1, Integrator4/1
  Integrator4/1 -> Sum3/2
  Sum3/1 -> Gain3/1
  Gain4/1 -> Sum3/1

== system transientStability_R14SP1/PSS/frequency_input_PSS /delay ==
  Vin : Inport
  Gain : Gain  Gain=1./mpc.dynamicdata.gen_pssParameters.pss_freq_signalParameters.Td1_freq  SaturateOnIntegerOverflow=on
  Integrator2 : Integrator
  Sum : Sum  Inputs=+-  SaturateOnIntegerOverflow=on  InputSameDT=on
  Out1 : Outport
  wires:
  Gain/1 -> Integrator2/1
  Sum/1 -> Gain/1
  Integrator2/1 -> Out1/1, Sum/2
  Vin/1 -> Sum/1

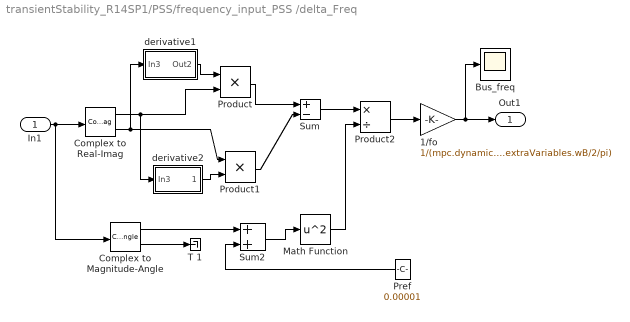
== system transientStability_R14SP1/PSS/frequency_input_PSS /delta_Freq ==
  In1 : Inport
  1/fo : Gain  Gain=1/(mpc.dynamicdata.extraVariables.wB/2/pi)  SaturateOnIntegerOverflow=on
  Bus_freq : Scope
      settings: TimeRange=3  MaxDataPoints=5000  SaveToWorkspace=off  SaveName=ScopeData  YMin=-0.4  YMax=0.5  SampleTime=-1
  Complex to Magnitude-Angle : ComplexToMagnitudeAngle
  Complex to Real-Imag : ComplexToRealImag
  Math Function : Math  Operator=square  SaturateOnIntegerOverflow=on
  Pref : Constant  Orientation=left  Value=0.00001
  Product : Product  SaturateOnIntegerOverflow=on  RndMeth=Zero  InputSameDT=on
  Product1 : Product  SaturateOnIntegerOverflow=on  RndMeth=Zero  InputSameDT=on
  Product2 : Product  Inputs=*/  SaturateOnIntegerOverflow=on  RndMeth=Zero  InputSameDT=on
  Sum : Sum  Inputs=+-  SaturateOnIntegerOverflow=on  InputSameDT=on
  Sum2 : Sum  SaturateOnIntegerOverflow=on  InputSameDT=on
  T 1 : Terminator
  derivative1 : Subsystem
  derivative2 : Subsystem
  Out1 : Outport
  wires:
  Complex to Real-Imag/1 -> Product/2, derivative2/1(In3)
  derivative1/1(Out2) -> Product/1
  Pref/1 -> Sum2/2
  Sum2/1 -> Math Function/1
  Complex to Magnitude-Angle/1 -> Sum2/1
  Product/1 -> Sum/1
  Product1/1 -> Sum/2
  Sum/1 -> Product2/1
  Math Function/1 -> Product2/2
  Complex to Real-Imag/2 -> Product1/1, derivative1/1(In3)
  derivative2/1(Out2) -> Product1/2
  Complex to Magnitude-Angle/2 -> T 1/1
  In1/1 -> Complex to Real-Imag/1, Complex to Magnitude-Angle/1
  Product2/1 -> 1/fo/1
  1/fo/1 -> Out1/1, Bus_freq/1

== system transientStability_R14SP1/STATIC LOADS/delta_Freq/derivative1 ==
  In3 : Inport
  1/1+s*Tf : Subsystem
  1/Tf : Gain  Gain=[1./0.02]/2/pi  SaturateOnIntegerOverflow=on
  Sum6 : Sum  Inputs=+-  SaturateOnIntegerOverflow=on  InputSameDT=on
  Out2 : Outport
  wires:
  1/Tf/1 -> Out2/1
  Sum6/1 -> 1/Tf/1
  1/1+s*Tf/1(Out1) -> Sum6/2
  In3/1 -> Sum6/1, 1/1+s*Tf/1(In1)

== system transientStability_R14SP1/STATIC LOADS/delta_Freq/derivative2 ==
  In3 : Inport
  1/1+s*Tf : Subsystem
  1/Tf : Gain  Gain=[1./0.02]/2/pi  SaturateOnIntegerOverflow=on
  Sum6 : Sum  Inputs=+-  SaturateOnIntegerOverflow=on  InputSameDT=on
  Out2 : Outport
  wires:
  In3/1 -> 1/1+s*Tf/1(In1), Sum6/1
  1/1+s*Tf/1(Out1) -> Sum6/2
  Sum6/1 -> 1/Tf/1
  1/Tf/1 -> Out2/1

== system transientStability_R14SP1/Turbine  system/Non Reheat Steam Turbine/DEMUXg2 ==
  In1 : Inport
  Dummy Zeros : Constant  Value=zeros(1,mpc.dynamicdata.extraVariables.nb-size(mpc.dynamicdata.turb_nrst,1))
  Mux1 : Mux  Inputs="[mpc.dynamicdata.extraVariables.nb-size(mpc.dynamicdata.turb_nrst,1)  size(mpc.dynamicdata.turb_nrst,1)]"
  Selector4 : Selector  InputPortWidth=mpc.dynamicdata.extraVariables.nb
  Out1 : Outport
  wires:
  In1/1 -> Mux1/2
  Selector4/1 -> Out1/1
  Dummy Zeros/1 -> Mux1/1
  Mux1/1 -> Selector4/1

== system transientStability_R14SP1/Turbine  system/Non Reheat Steam Turbine/Governer ==
  dWB : Inport
  Constant : Constant  Value=mpc.dynamicdata.gen_turbineParameters.NonReheat_turbineParameters.Pgv_nrt0
  Gain : Gain  Gain=1-mpc.dynamicdata.gen_turbineParameters.NonReheat_turbineParameters.T2_nrt./mpc.dynamicdata.gen_turbineParameters.NonReheat_turbineParameters.T1_nrt  SaturateOnIntegerOverflow=on
  Gain1 : Gain  Gain=1./mpc.dynamicdata.gen_turbineParameters.NonReheat_turbineParameters.T1_nrt  SaturateOnIntegerOverflow=on
  Gain2 : Gain  Gain=mpc.dynamicdata.gen_turbineParameters.NonReheat_turbineParameters.T2_nrt./mpc.dynamicdata.gen_turbineParameters.NonReheat_turbineParameters.T1_nrt  SaturateOnIntegerOverflow=on
  Gain3 : Gain  Gain=mpc.dynamicdata.gen_turbineParameters.NonReheat_turbineParameters.K_nrt  SaturateOnIntegerOverflow=on
  Gain4 : Gain  Gain=1./mpc.dynamicdata.gen_turbineParameters.NonReheat_turbineParameters.T3_nrt  SaturateOnIntegerOverflow=on
  Integrator : Integrator
  Integrator1 : Integrator  InitialCondition=mpc.dynamicdata.gen_turbineParameters.NonReheat_turbineParameters.Pgv_nrt0  LimitOutput=on  UpperSaturationLimit=mpc.dynamicdata.gen_turbineParameters.NonReheat_turbineParameters.Pgv_nrt_max.*mpc.dynamicdata.gen_turbineParameters.NonReheat_turbineParameters.Pgv_nrt0  LowerSaturationLimit=mpc.dynamicdata.gen_turbineParameters.NonReheat_turbineParameters.Pgv_nrt_min.*mpc.dynamicdata.gen_turbineParameters.NonReheat_turbineParameters.Pgv_nrt0
  Sum : Sum  Inputs=+-  SaturateOnIntegerOverflow=on  InputSameDT=on
  Sum1 : Sum  SaturateOnIntegerOverflow=on  InputSameDT=on
  Sum3 : Sum  Inputs=+--  SaturateOnIntegerOverflow=on  InputSameDT=on
  Pgv : Outport
  wires:
  Sum/1 -> Gain1/1
  Gain/1 -> Sum/1
  Integrator/1 -> Sum1/1, Sum/2
  Gain2/1 -> Sum1/2
  Gain1/1 -> Integrator/1
  Sum1/1 -> Gain3/1
  Sum3/1 -> Gain4/1
  Gain4/1 -> Integrator1/1
  Integrator1/1 -> Sum3/3, Pgv/1
  Gain3/1 -> Sum3/2
  Constant/1 -> Sum3/1
  dWB/1 -> Gain/1, Gain2/1

== system transientStability_R14SP1/Turbine  system/Non Reheat Steam Turbine/Nonreheat ==
  Pgv : Inport
  Gain : Gain  Gain=1./mpc.dynamicdata.gen_turbineParameters.NonReheat_turbineParameters.Tch_nrt  SaturateOnIntegerOverflow=on
  Integrator : Integrator  InitialCondition=mpc.dynamicdata.gen_turbineParameters.NonReheat_turbineParameters.Pgv_nrt0
  Sum : Sum  Inputs=|+-  SaturateOnIntegerOverflow=on  InputSameDT=on
  Tm : Outport
  wires:
  Gain/1 -> Integrator/1
  Sum/1 -> Gain/1
  Integrator/1 -> Sum/2, Tm/1
  Pgv/1 -> Sum/1

== system transientStability_R14SP1/Turbine  system/Non Reheat Steam Turbine/Select-Turbine ==
  in_1 : Inport
  in_2 : Inport  Port=2
  Switch : Switch  Threshold=1  SaturateOnIntegerOverflow=on  InputSameDT=on
  zeros : Constant  Value=zeros(1,mpc.dynamicdata.extraVariables.nb)
  out_1 : Outport  InitialOutput=0
  wires:
  Switch/1 -> out_1/1
  in_1/1 -> Switch/2
  in_2/1 -> Switch/3
  zeros/1 -> Switch/1

== system transientStability_R14SP1/Turbine  system/Sped Gov_Hydro Turbine/DEMUXg2 ==
  In1 : Inport
  Dummy Zeros : Constant  Value=zeros(1,mpc.dynamicdata.extraVariables.nb-size(mpc.dynamicdata.turb_hydro,1))
  Mux1 : Mux  Inputs="[mpc.dynamicdata.extraVariables.nb-size(mpc.dynamicdata.turb_hydro,1)  size(mpc.dynamicdata.turb_hydro,1)]"
  Selector4 : Selector  InputPortWidth=mpc.dynamicdata.extraVariables.nb
  Out1 : Outport
  wires:
  Mux1/1 -> Selector4/1
  Dummy Zeros/1 -> Mux1/1
  Selector4/1 -> Out1/1
  In1/1 -> Mux1/2

== system transientStability_R14SP1/Turbine  system/Sped Gov_Hydro Turbine/Governer ==
  del WB : Inport
  Constant : Constant  Value=mpc.dynamicdata.gen_turbineParameters.hydro_turbineParameters.Pgv_ht0
  Gain : Gain  Gain=1-mpc.dynamicdata.gen_turbineParameters.hydro_turbineParameters.T2_ht./mpc.dynamicdata.gen_turbineParameters.hydro_turbineParameters.T1_ht  SaturateOnIntegerOverflow=on
  Gain1 : Gain  Gain=1./mpc.dynamicdata.gen_turbineParameters.hydro_turbineParameters.T1_ht  SaturateOnIntegerOverflow=on
  Gain2 : Gain  Gain=mpc.dynamicdata.gen_turbineParameters.hydro_turbineParameters.T2_ht./mpc.dynamicdata.gen_turbineParameters.hydro_turbineParameters.T1_ht  SaturateOnIntegerOverflow=on
  Gain3 : Gain  Gain=mpc.dynamicdata.gen_turbineParameters.hydro_turbineParameters.K_ht  SaturateOnIntegerOverflow=on
  Gain4 : Gain  Gain=1./mpc.dynamicdata.gen_turbineParameters.hydro_turbineParameters.T3_ht  SaturateOnIntegerOverflow=on
  Integrator : Integrator
  Integrator1 : Integrator
  Saturation : Saturate  UpperLimit=mpc.dynamicdata.gen_turbineParameters.hydro_turbineParameters.Pgv_ht_max.*mpc.dynamicdata.gen_turbineParameters.hydro_turbineParameters.Pgv_ht0  LowerLimit=mpc.dynamicdata.gen_turbineParameters.hydro_turbineParameters.Pgv_ht_min.*mpc.dynamicdata.gen_turbineParameters.hydro_turbineParameters.Pgv_ht0
  Sum : Sum  Inputs=+-  SaturateOnIntegerOverflow=on  InputSameDT=on
  Sum1 : Sum  SaturateOnIntegerOverflow=on  InputSameDT=on
  Sum3 : Sum  Inputs=+-  SaturateOnIntegerOverflow=on  InputSameDT=on
  Sum4 : Sum  Inputs=+-  SaturateOnIntegerOverflow=on  InputSameDT=on
  Pgv : Outport
  wires:
  Sum/1 -> Gain1/1
  Gain/1 -> Sum/1
  Integrator/1 -> Sum/2, Sum1/1
  Gain2/1 -> Sum1/2
  Gain1/1 -> Integrator/1
  del WB/1 -> Gain2/1, Gain/1
  Sum1/1 -> Gain3/1
  Gain3/1 -> Sum3/1
  Sum3/1 -> Gain4/1
  Gain4/1 -> Integrator1/1
  Integrator1/1 -> Sum4/2, Sum3/2
  Constant/1 -> Sum4/1
  Sum4/1 -> Saturation/1
  Saturation/1 -> Pgv/1

== system transientStability_R14SP1/Turbine  system/Sped Gov_Hydro Turbine/HydroTurbine ==
  Pgv : Inport
  Gain : Gain  Gain=1-(-mpc.dynamicdata.gen_turbineParameters.hydro_turbineParameters.T_wht)./(0.5*mpc.dynamicdata.gen_turbineParameters.hydro_turbineParameters.T_wht)  SaturateOnIntegerOverflow=on
  Gain1 : Gain  Gain=1./(0.5*mpc.dynamicdata.gen_turbineParameters.hydro_turbineParameters.T_wht)  SaturateOnIntegerOverflow=on
  Gain2 : Gain  Gain=-mpc.dynamicdata.gen_turbineParameters.hydro_turbineParameters.T_wht./(0.5*mpc.dynamicdata.gen_turbineParameters.hydro_turbineParameters.T_wht)  SaturateOnIntegerOverflow=on
  Integrator : Integrator  InitialCondition=mpc.dynamicdata.gen_turbineParameters.hydro_turbineParameters.Tgr_ht0
  Sum : Sum  Inputs=+-  SaturateOnIntegerOverflow=on  InputSameDT=on
  Sum1 : Sum  SaturateOnIntegerOverflow=on  InputSameDT=on
  Tm : Outport
  wires:
  Sum1/1 -> Tm/1
  Gain1/1 -> Integrator/1
  Pgv/1 -> Gain2/1, Gain/1
  Gain2/1 -> Sum1/2
  Integrator/1 -> Sum/2, Sum1/1
  Gain/1 -> Sum/1
  Sum/1 -> Gain1/1

== system transientStability_R14SP1/Turbine  system/Sped Gov_Hydro Turbine/Select-Turbine ==
  in_1 : Inport
  in_2 : Inport  Port=2
  Switch : Switch  Threshold=1  SaturateOnIntegerOverflow=on  InputSameDT=on
  zeros : Constant  Value=zeros(1,mpc.dynamicdata.extraVariables.nb)
  out_1 : Outport  InitialOutput=0
  wires:
  Switch/1 -> out_1/1
  in_1/1 -> Switch/2
  in_2/1 -> Switch/3
  zeros/1 -> Switch/1

== system transientStability_R14SP1/Turbine  system/Speed Gov. Reheat Steam  Turbine/DEMUXg2 ==
  In1 : Inport
  Dummy Zeros : Constant  Value=zeros(1,mpc.dynamicdata.extraVariables.nb-size(mpc.dynamicdata.turb_rhst,1))
  Mux1 : Mux  Inputs="[mpc.dynamicdata.extraVariables.nb-size(mpc.dynamicdata.turb_rhst,1)  size(mpc.dynamicdata.turb_rhst,1)]"
  Selector4 : Selector  InputPortWidth=mpc.dynamicdata.extraVariables.nb
  Out1 : Outport
  wires:
  In1/1 -> Mux1/2
  Selector4/1 -> Out1/1
  Dummy Zeros/1 -> Mux1/1
  Mux1/1 -> Selector4/1

== system transientStability_R14SP1/Turbine  system/Speed Gov. Reheat Steam  Turbine/Governer ==
  dWB : Inport
  Constant : Constant  Value=mpc.dynamicdata.gen_turbineParameters.Reheat_turbineParameters.Pgv_rht0
  Gain : Gain  Gain=1-mpc.dynamicdata.gen_turbineParameters.Reheat_turbineParameters.T2_rht./mpc.dynamicdata.gen_turbineParameters.Reheat_turbineParameters.T1_rht  SaturateOnIntegerOverflow=on
  Gain1 : Gain  Gain=1./mpc.dynamicdata.gen_turbineParameters.Reheat_turbineParameters.T1_rht  SaturateOnIntegerOverflow=on
  Gain2 : Gain  Gain=mpc.dynamicdata.gen_turbineParameters.Reheat_turbineParameters.T2_rht./mpc.dynamicdata.gen_turbineParameters.Reheat_turbineParameters.T1_rht  SaturateOnIntegerOverflow=on
  Gain3 : Gain  Gain=mpc.dynamicdata.gen_turbineParameters.Reheat_turbineParameters.K_rht  SaturateOnIntegerOverflow=on
  Gain4 : Gain  Gain=1./mpc.dynamicdata.gen_turbineParameters.Reheat_turbineParameters.T3_rht  SaturateOnIntegerOverflow=on
  Integrator : Integrator
  Integrator1 : Integrator  InitialCondition=mpc.dynamicdata.gen_turbineParameters.Reheat_turbineParameters.Pgv_rht0  LimitOutput=on  UpperSaturationLimit=mpc.dynamicdata.gen_turbineParameters.Reheat_turbineParameters.Pgv_rht_max.*mpc.dynamicdata.gen_turbineParameters.Reheat_turbineParameters.Pgv_rht0  LowerSaturationLimit=mpc.dynamicdata.gen_turbineParameters.Reheat_turbineParameters.Pgv_rht_min.*mpc.dynamicdata.gen_turbineParameters.Reheat_turbineParameters.Pgv_rht0
  Sum : Sum  Inputs=+-  SaturateOnIntegerOverflow=on  InputSameDT=on
  Sum1 : Sum  SaturateOnIntegerOverflow=on  InputSameDT=on
  Sum3 : Sum  Inputs=+--  SaturateOnIntegerOverflow=on  InputSameDT=on
  Pgv : Outport
  wires:
  Sum/1 -> Gain1/1
  Gain/1 -> Sum/1
  Integrator/1 -> Sum1/1, Sum/2
  Gain2/1 -> Sum1/2
  Gain1/1 -> Integrator/1
  Sum1/1 -> Gain3/1
  Sum3/1 -> Gain4/1
  Gain4/1 -> Integrator1/1
  Integrator1/1 -> Sum3/3, Pgv/1
  Gain3/1 -> Sum3/2
  Constant/1 -> Sum3/1
  dWB/1 -> Gain/1, Gain2/1

== system transientStability_R14SP1/Turbine  system/Speed Gov. Reheat Steam  Turbine/Reheat ==
  Pgv : Inport
  Crossover : Subsystem
  Gain3 : Gain  Gain=mpc.dynamicdata.gen_turbineParameters.Reheat_turbineParameters.FHP_rht  SaturateOnIntegerOverflow=on
  Gain4 : Gain  Gain=mpc.dynamicdata.gen_turbineParameters.Reheat_turbineParameters.FIP_rht  SaturateOnIntegerOverflow=on
  Gain5 : Gain  Gain=mpc.dynamicdata.gen_turbineParameters.Reheat_turbineParameters.FLP_rht  SaturateOnIntegerOverflow=on
  Reheater : Subsystem
  St.Chest : Subsystem
  Sum5 : Sum  Inputs=+++  SaturateOnIntegerOverflow=on  InputSameDT=on
  Pm : Outport
  wires:
  Crossover/1(Out1) -> Gain5/1
  Reheater/1(Out1) -> Crossover/1(In1), Gain4/1
  St.Chest/1(Out1) -> Reheater/1(In1), Gain3/1
  Gain5/1 -> Sum5/3
  Gain4/1 -> Sum5/2
  Gain3/1 -> Sum5/1
  Sum5/1 -> Pm/1
  Pgv/1 -> St.Chest/1(In1)

== system transientStability_R14SP1/Turbine  system/Speed Gov. Reheat Steam  Turbine/Select-Turbine ==
  in_1 : Inport
  in_2 : Inport  Port=2
  Switch : Switch  Threshold=1  SaturateOnIntegerOverflow=on  InputSameDT=on
  zeros : Constant  Value=zeros(1,mpc.dynamicdata.extraVariables.nb)
  out_1 : Outport  InitialOutput=0
  wires:
  Switch/1 -> out_1/1
  in_1/1 -> Switch/2
  in_2/1 -> Switch/3
  zeros/1 -> Switch/1

== system transientStability_R14SP1/Excitation system/Exciter_AC1A /Exciter AC1A/ESS ==
  vfe : Inport
  Gain3 : Gain  Gain=1./mpc.dynamicdata.gen_exciterParameters.AC1A_exciterParameters.TF_AC1A  SaturateOnIntegerOverflow=on
  Gain4 : Gain  Gain=mpc.dynamicdata.gen_exciterParameters.AC1A_exciterParameters.KF_AC1A  SaturateOnIntegerOverflow=on
  Integrator4 : Integrator  InitialCondition=mpc.dynamicdata.gen_exciterParameters.AC1A_exciterParameters.Fst0_AC1A
  Sum3 : Sum  Inputs=+-  SaturateOnIntegerOverflow=on  InputSameDT=on
  VF1 : Outport  Orientation=up
  wires:
  vfe/1 -> Gain4/1
  Sum3/1 -> Gain3/1
  Gain4/1 -> Sum3/1
  Gain3/1 -> Integrator4/1, VF1/1
  Integrator4/1 -> Sum3/2

== system transientStability_R14SP1/Excitation system/Exciter_AC1A /Exciter AC1A/Regulator ==
  Vin : Inport
  Gain : Gain  Gain=1./mpc.dynamicdata.gen_exciterParameters.AC1A_exciterParameters.TA_AC1A  SaturateOnIntegerOverflow=on
  Gain1 : Gain  Gain=mpc.dynamicdata.gen_exciterParameters.AC1A_exciterParameters.kA_AC1A  SaturateOnIntegerOverflow=on
  Integrator2 : Integrator  InitialCondition=mpc.dynamicdata.gen_exciterParameters.AC1A_exciterParameters.VR0_AC1A  LimitOutput=on  UpperSaturationLimit=mpc.dynamicdata.gen_exciterParameters.AC1A_exciterParameters.VAmax_AC1A  LowerSaturationLimit=mpc.dynamicdata.gen_exciterParameters.AC1A_exciterParameters.VAmin_AC1A
  Sum : Sum  Inputs=+-  SaturateOnIntegerOverflow=on  InputSameDT=on
  VR : Outport
  wires:
  Sum/1 -> Gain/1
  Integrator2/1 -> VR/1, Sum/2
  Gain1/1 -> Sum/1
  Gain/1 -> Integrator2/1
  Vin/1 -> Gain1/1

== system transientStability_R14SP1/Excitation system/Exciter_AC1A /Exciter AC1A/Subsystem1 ==
  VE : Inport
  IFD : Inport  Port=2
  Rec-Reg Curve : Subsystem
  Saturation : Subsystem
  FEX : Outport
  VFE : Outport  Port=2
  wires:
  Rec-Reg Curve/1(Fex) -> FEX/1
  Saturation/1(Vfe) -> VFE/1
  VE/1 -> Saturation/1(Ve), Rec-Reg Curve/2(Ve)
  IFD/1 -> Saturation/2(Ifd), Rec-Reg Curve/1(Ifd)

== system transientStability_R14SP1/Excitation system/Exciter_AC1A /Exciter AC1A/TGR ==
  Ver : Inport
  Gain3 : Gain  Gain=1./mpc.dynamicdata.gen_exciterParameters.AC1A_exciterParameters.TB_AC1A  SaturateOnIntegerOverflow=on
  Gain4 : Gain  Gain=mpc.dynamicdata.gen_exciterParameters.AC1A_exciterParameters.TC_AC1A./mpc.dynamicdata.gen_exciterParameters.AC1A_exciterParameters.TB_AC1A  SaturateOnIntegerOverflow=on
  Gain5 : Gain  Gain=1-mpc.dynamicdata.gen_exciterParameters.AC1A_exciterParameters.TC_AC1A./mpc.dynamicdata.gen_exciterParameters.AC1A_exciterParameters.TB_AC1A  SaturateOnIntegerOverflow=on
  Integrator4 : Integrator  InitialCondition=mpc.dynamicdata.gen_exciterParameters.AC1A_exciterParameters.Tgr0_AC1A
  Sum3 : Sum  SaturateOnIntegerOverflow=on  InputSameDT=on
  Sum4 : Sum  Inputs=+-  SaturateOnIntegerOverflow=on  InputSameDT=on
  Vtgr : Outport
  wires:
  Sum3/1 -> Vtgr/1
  Gain4/1 -> Sum3/2
  Integrator4/1 -> Sum3/1, Sum4/2
  Sum4/1 -> Gain3/1
  Gain5/1 -> Sum4/1
  Gain3/1 -> Integrator4/1
  Ver/1 -> Gain4/1, Gain5/1

== system transientStability_R14SP1/Excitation system/Exciter_AC1A /Exciter AC1A/delay1 ==
  Vin : Inport
  Gain : Gain  Gain=1./mpc.dynamicdata.gen_exciterParameters.AC1A_exciterParameters.Tr_AC1A  SaturateOnIntegerOverflow=on
  Integrator2 : Integrator  InitialCondition=mpc.dynamicdata.extraVariables.lfl(mpc.dynamicdata.exc_AC1A(:,1),2)
  Sum : Sum  Inputs=+-  SaturateOnIntegerOverflow=on  InputSameDT=on
  Out1 : Outport
  wires:
  Vin/1 -> Sum/1
  Integrator2/1 -> Sum/2, Out1/1
  Sum/1 -> Gain/1
  Gain/1 -> Integrator2/1

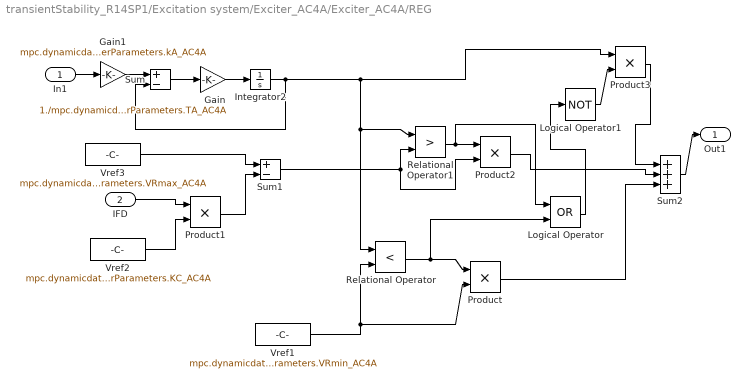
== system transientStability_R14SP1/Excitation system/Exciter_AC4A/Exciter_AC4A/REG ==
  In1 : Inport
  IFD : Inport  Port=2
  Gain : Gain  Gain=1./mpc.dynamicdata.gen_exciterParameters.AC4A_exciterParameters.TA_AC4A  SaturateOnIntegerOverflow=on
  Gain1 : Gain  Gain=mpc.dynamicdata.gen_exciterParameters.AC4A_exciterParameters.kA_AC4A  SaturateOnIntegerOverflow=on
  Integrator2 : Integrator  InitialCondition=mpc.dynamicdata.gen_exciterParameters.AC4A_exciterParameters.Efd0_AC4A
  Logical Operator : Logic  Operator=OR
  Logical Operator1 : Logic  Operator=NOT
  Product{,1..3} (4 alike) : Product  SaturateOnIntegerOverflow=on  RndMeth=Zero  InputSameDT=on
  Relational Operator : RelationalOperator  Operator=<  InputSameDT=on
  Relational Operator1 : RelationalOperator  Operator=>  InputSameDT=on
  Sum : Sum  Inputs=+-  SaturateOnIntegerOverflow=on  InputSameDT=on
  Sum1 : Sum  Inputs=+-  SaturateOnIntegerOverflow=on  InputSameDT=on
  Sum2 : Sum  Inputs=+++  SaturateOnIntegerOverflow=on  InputSameDT=on
  Vref1 : Constant  Value=mpc.dynamicdata.gen_exciterParameters.AC4A_exciterParameters.VRmin_AC4A
  Vref2 : Constant  Value=mpc.dynamicdata.gen_exciterParameters.AC4A_exciterParameters.KC_AC4A
  Vref3 : Constant  Value=mpc.dynamicdata.gen_exciterParameters.AC4A_exciterParameters.VRmax_AC4A
  Out1 : Outport
  wires:
  In1/1 -> Gain1/1
  Gain1/1 -> Sum/1
  Sum/1 -> Gain/1
  Integrator2/1 -> Sum/2, Relational Operator/1, Relational Operator1/1, Product3/1
  Gain/1 -> Integrator2/1
  Vref1/1 -> Relational Operator/2, Product/2
  Vref2/1 -> Product1/2
  IFD/1 -> Product1/1
  Vref3/1 -> Sum1/1
  Product1/1 -> Sum1/2
  Sum1/1 -> Relational Operator1/2, Product2/2
  Product2/1 -> Sum2/2
  Product/1 -> Sum2/3
  Relational Operator/1 -> Product/1, Logical Operator/2
  Relational Operator1/1 -> Product2/1, Logical Operator/1
  Logical Operator/1 -> Logical Operator1/1
  Logical Operator1/1 -> Product3/2
  Product3/1 -> Sum2/1
  Sum2/1 -> Out1/1

== system transientStability_R14SP1/Excitation system/Exciter_AC4A/Exciter_AC4A/TGR ==
  Ver : Inport
  Gain3 : Gain  Gain=1./mpc.dynamicdata.gen_exciterParameters.AC4A_exciterParameters.TB_AC4A  SaturateOnIntegerOverflow=on
  Gain4 : Gain  Gain=mpc.dynamicdata.gen_exciterParameters.AC4A_exciterParameters.TC_AC4A./mpc.dynamicdata.gen_exciterParameters.AC4A_exciterParameters.TB_AC4A  SaturateOnIntegerOverflow=on
  Gain5 : Gain  Gain=1-mpc.dynamicdata.gen_exciterParameters.AC4A_exciterParameters.TC_AC4A./mpc.dynamicdata.gen_exciterParameters.AC4A_exciterParameters.TB_AC4A  SaturateOnIntegerOverflow=on
  Integrator4 : Integrator  InitialCondition=mpc.dynamicdata.gen_exciterParameters.AC4A_exciterParameters.Tgr0_AC4A
  Sum3 : Sum  SaturateOnIntegerOverflow=on  InputSameDT=on
  Sum4 : Sum  Inputs=+-  SaturateOnIntegerOverflow=on  InputSameDT=on
  V3 : Outport
  wires:
  Gain5/1 -> Sum4/1
  Sum4/1 -> Gain3/1
  Gain3/1 -> Integrator4/1
  Integrator4/1 -> Sum4/2, Sum3/1
  Gain4/1 -> Sum3/2
  Ver/1 -> Gain5/1, Gain4/1
  Sum3/1 -> V3/1

== system transientStability_R14SP1/Excitation system/Exciter_AC4A/Exciter_AC4A/delay1 ==
  Vin : Inport
  Gain : Gain  Gain=1./mpc.dynamicdata.gen_exciterParameters.AC4A_exciterParameters.Tr_AC4A  SaturateOnIntegerOverflow=on
  Integrator2 : Integrator  InitialCondition=mpc.dynamicdata.extraVariables.lfl(mpc.dynamicdata.exc_AC4A(:,1),2)
  Sum : Sum  Inputs=+-  SaturateOnIntegerOverflow=on  InputSameDT=on
  Out1 : Outport
  wires:
  Vin/1 -> Sum/1
  Integrator2/1 -> Sum/2, Out1/1
  Sum/1 -> Gain/1
  Gain/1 -> Integrator2/1

== system transientStability_R14SP1/Excitation system/Exciter_DC1A/Subsystem/ESS ==
  Efd : Inport
  Gain3 : Gain  Gain=1./mpc.dynamicdata.gen_exciterParameters.DC1A_exciterParameters.TF_DC1A  SaturateOnIntegerOverflow=on
  Gain4 : Gain  Gain=mpc.dynamicdata.gen_exciterParameters.DC1A_exciterParameters.KF_DC1A  SaturateOnIntegerOverflow=on
  Integrator4 : Integrator  InitialCondition=mpc.dynamicdata.gen_exciterParameters.DC1A_exciterParameters.Fst0_DC1A
  Sum3 : Sum  Inputs=+-  SaturateOnIntegerOverflow=on  InputSameDT=on
  VF : Outport  Orientation=up
  wires:
  Gain4/1 -> Sum3/1
  Sum3/1 -> Gain3/1
  Integrator4/1 -> Sum3/2
  Gain3/1 -> Integrator4/1, VF/1
  Efd/1 -> Gain4/1

== system transientStability_R14SP1/Excitation system/Exciter_DC1A/Subsystem/Regulator ==
  Vin : Inport
  Gain : Gain  Gain=1./mpc.dynamicdata.gen_exciterParameters.DC1A_exciterParameters.TA_DC1A  SaturateOnIntegerOverflow=on
  Gain1 : Gain  Gain=mpc.dynamicdata.gen_exciterParameters.DC1A_exciterParameters.KA_DC1A  SaturateOnIntegerOverflow=on
  Integrator2 : Integrator  InitialCondition=mpc.dynamicdata.gen_exciterParameters.DC1A_exciterParameters.VR0_DC1A  LimitOutput=on  UpperSaturationLimit=mpc.dynamicdata.gen_exciterParameters.DC1A_exciterParameters.VRmax_DC1A  LowerSaturationLimit=mpc.dynamicdata.gen_exciterParameters.DC1A_exciterParameters.VRmin_DC1A
  Sum : Sum  Inputs=+-  SaturateOnIntegerOverflow=on  InputSameDT=on
  Out1 : Outport
  wires:
  Gain1/1 -> Sum/1
  Integrator2/1 -> Sum/2, Out1/1
  Sum/1 -> Gain/1
  Gain/1 -> Integrator2/1
  Vin/1 -> Gain1/1
